simulink model "closed_loop"  (R2020a)
settings: Solver=ode45  StartTime=0.0  StopTime=10.0  RelTol=1e-3
values from neighbouring files (symbols this model uses):
  K = K8    [main.m]
  Kd = 1    [main.m]
  p = 4*N(i,j)-R1p    [h2AG.m]    (also in h2AS.m = 4*ns-R1p; parameters.mat = ; set_parameters.m = para)
undefined symbols (not defined in the file or in its folder): magnitude, sigbuilder_block
settings Model: Creator=mecsh  LastModifiedBy=mecsh

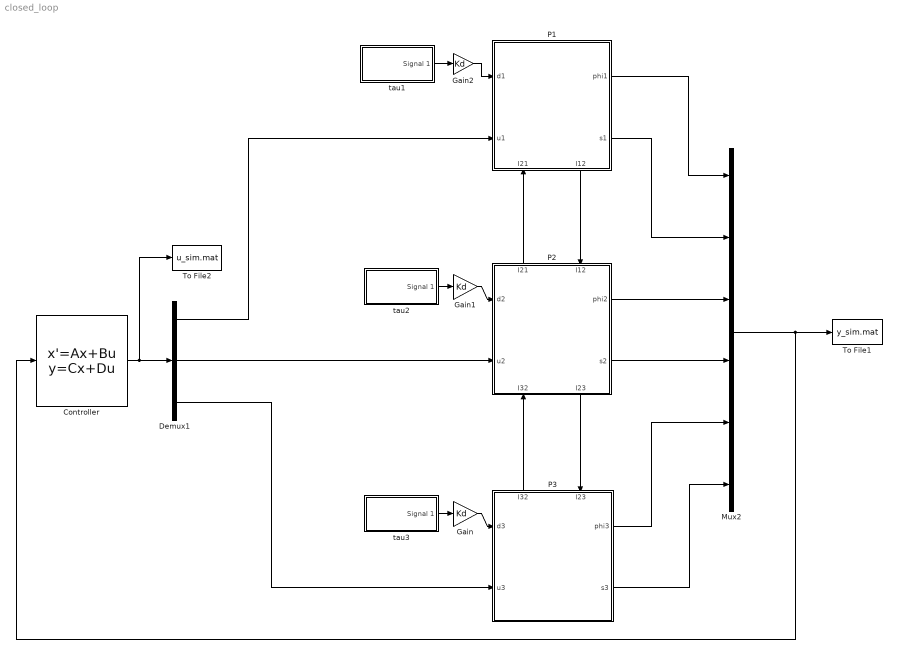
== system closed_loop ==
  Controller : StateSpace  A=K.A  B=K.B  C=K.C  D=K.D  InitialCondition=0
  Demux1 : Demux  Outputs=3
  Gain : Gain  Gain=Kd
  Gain1 : Gain  Gain=Kd
  Gain2 : Gain  Gain=Kd
  Mux2 : Mux  Inputs=6
  P1 : Subsystem
      settings: PortSchema="{\"entries\":[{\"content\":{\"sides\":[{\"content\":{\"connectorIds\":[\"In1\",\"In2\"]},\"type\":\"ConnectorPlacement.EquallySpacedRectSide\",\"uuid\":\"8ecf2bd6-8dd7-4624-a6b6-31e540f77a47\"},{\"content\":{\"connectorIds\":[\"Out1\",\"Out2\"],\"side\":\"RIGHT\"},\"type\":\"ConnectorPlacement.EquallySpacedRectSide\",\"uuid\":\"8430024e-b75d-4fb2-99a2-0065abf52074\"},{\"content\":{\"connectorIds\":[],\"side\":\"TOP\"},\"type\":\"ConnectorPlacement.EquallySpacedRectSide\",\"uuid\":\"c038c5bf-c588-4120-bde9-e57e7985113f\"},{\"content\":{\"connectorIds\":[\"In3\",\"Out3\"],\"side\":\"BOTTOM\"},\"type\":\"ConnectorPlacement.EquallySpacedRectSide\",\"uuid\":\"e08f6579-8c34-4bda-96ff-48e678e21df1\"}]},\"type\":\"ConnectorPlacement.EquallySpacedConnector\",\"uuid\":\"e152476a-752c-407e-9d79-b57d158a90de\"}],\"packageUris\":[\"http://schema.mathworks.com/mf0/Connector/19700101\"],\"version\":\"1.0\"}"
  P2 : Subsystem
      settings: PortSchema="{\"entries\":[{\"content\":{\"sides\":[{\"content\":{\"connectorIds\":[\"In1\",\"In2\"]},\"type\":\"ConnectorPlacement.EquallySpacedRectSide\",\"uuid\":\"4bcbf91d-3e1f-4b18-9cf2-1c48cd989a02\"},{\"content\":{\"connectorIds\":[\"Out1\",\"Out2\"],\"side\":\"RIGHT\"},\"type\":\"ConnectorPlacement.EquallySpacedRectSide\",\"uuid\":\"817b564b-dbb4-4a38-a63d-192f41fddb5e\"},{\"content\":{\"connectorIds\":[\"Out4\",\"In3\"],\"side\":\"TOP\"},\"type\":\"ConnectorPlacement.EquallySpacedRectSide\",\"uuid\":\"a66c876f-ee47-4f3c-90a0-c8c684866f46\"},{\"content\":{\"connectorIds\":[\"In4\",\"Out3\"],\"side\":\"BOTTOM\"},\"type\":\"ConnectorPlacement.EquallySpacedRectSide\",\"uuid\":\"ae0f9748-517d-4fb0-b861-7e671e2401a3\"}]},\"type\":\"ConnectorPlacement.EquallySpacedConnector\",\"uuid\":\"71628be4-01f7-4652-8912-34b5b1a2183b\"}],\"packageUris\":[\"http://schema.mathworks.com/mf0/Connector/19700101\"],\"version\":\"1.0\"}"
  P3 : Subsystem
      settings: PortSchema="{\"entries\":[{\"content\":{\"sides\":[{\"content\":{\"connectorIds\":[\"In1\",\"In2\"]},\"type\":\"ConnectorPlacement.EquallySpacedRectSide\",\"uuid\":\"4bcbf91d-3e1f-4b18-9cf2-1c48cd989a02\"},{\"content\":{\"connectorIds\":[\"Out1\",\"Out2\"],\"side\":\"RIGHT\"},\"type\":\"ConnectorPlacement.EquallySpacedRectSide\",\"uuid\":\"817b564b-dbb4-4a38-a63d-192f41fddb5e\"},{\"content\":{\"connectorIds\":[\"Out3\",\"In3\"],\"side\":\"TOP\"},\"type\":\"ConnectorPlacement.EquallySpacedRectSide\",\"uuid\":\"a66c876f-ee47-4f3c-90a0-c8c684866f46\"},{\"content\":{\"connectorIds\":[],\"side\":\"BOTTOM\"},\"type\":\"ConnectorPlacement.EquallySpacedRectSide\",\"uuid\":\"ae0f9748-517d-4fb0-b861-7e671e2401a3\"}]},\"type\":\"ConnectorPlacement.EquallySpacedConnector\",\"uuid\":\"71628be4-01f7-4652-8912-34b5b1a2183b\"}],\"packageUris\":[\"http://schema.mathworks.com/mf0/Connector/19700101\"],\"version\":\"1.0\"}"
  To File1 : ToFile  Filename=y_sim.mat  MatrixName=y_sim  SampleTime=0.01
  To File2 : ToFile  Filename=u_sim.mat  MatrixName=u_sim  SampleTime=0.01
  tau1 : Subsystem  Tag=STV Subsys  LoadFcn=sigbuilder_block('load');  StartFcn=sigbuilder_block('start');  StopFcn=sigbuilder_block('stop');  ClipboardFcn=sigbuilder_block('clipboard');  mask(Sigbuilder block){tuvar=[0:10]}
      mask help: Simulink:masks:SigbuilderBlock_MD
      mask init:
      | if ~strcmp(get_param(bdroot(gcbh),'SimulationStatus'),'stopped') tuvar = sigbuilder_block('maskInit'); end
      settings: CopyFcn=sigbuilder_block('copy');  DeleteFcn=sigbuilder_block('delete');  ModelCloseFcn=sigbuilder_block('modelClose');  PreSaveFcn=sigbuilder_block('preSave');  PauseFcn=sigbuilder_block('pause');  ContinueFcn=sigbuilder_block('continue');  NameChangeFcn=sigbuilder_block('namechange');  OpenFcn=sigbuilder_block('open',[437.6 199.2 550.4 400 ]);  CloseFcn=sigbuilder_block('close');
      mask Display: plot(0, 0, 100, 100,[2, 2, 32, 32, 2], [68, 8, 8, 68, 68],[32, 2], [38, 38], [32, 19, 2],[53, 60, 44], [32, 17, 17, 2],[16, 16, 31, 31]);txt = getActiveGroup(gcbh);text(2, 100, txt,'verticalAlignment', 'top');
  tau2 : Subsystem  Tag=STV Subsys  LoadFcn=sigbuilder_block('load');  StartFcn=sigbuilder_block('start');  StopFcn=sigbuilder_block('stop');  ClipboardFcn=sigbuilder_block('clipboard');  mask(Sigbuilder block){tuvar=[0:10]}
      mask help: Simulink:masks:SigbuilderBlock_MD
      mask init:
      | if ~strcmp(get_param(bdroot(gcbh),'SimulationStatus'),'stopped') tuvar = sigbuilder_block('maskInit'); end
      settings: CopyFcn=sigbuilder_block('copy');  DeleteFcn=sigbuilder_block('delete');  ModelCloseFcn=sigbuilder_block('modelClose');  PreSaveFcn=sigbuilder_block('preSave');  PauseFcn=sigbuilder_block('pause');  ContinueFcn=sigbuilder_block('continue');  NameChangeFcn=sigbuilder_block('namechange');  OpenFcn=sigbuilder_block('open',[437.6 199.2 550.4 400 ]);  CloseFcn=sigbuilder_block('close');
      mask Display: plot(0, 0, 100, 100,[2, 2, 32, 32, 2], [68, 8, 8, 68, 68],[32, 2], [38, 38], [32, 19, 2],[53, 60, 44], [32, 17, 17, 2],[16, 16, 31, 31]);txt = getActiveGroup(gcbh);text(2, 100, txt,'verticalAlignment', 'top');
  tau3 : Subsystem  Tag=STV Subsys  LoadFcn=sigbuilder_block('load');  StartFcn=sigbuilder_block('start');  StopFcn=sigbuilder_block('stop');  ClipboardFcn=sigbuilder_block('clipboard');  mask(Sigbuilder block){tuvar=[0:10]}
      mask help: Simulink:masks:SigbuilderBlock_MD
      mask init:
      | if ~strcmp(get_param(bdroot(gcbh),'SimulationStatus'),'stopped') tuvar = sigbuilder_block('maskInit'); end
      settings: CopyFcn=sigbuilder_block('copy');  DeleteFcn=sigbuilder_block('delete');  ModelCloseFcn=sigbuilder_block('modelClose');  PreSaveFcn=sigbuilder_block('preSave');  PauseFcn=sigbuilder_block('pause');  ContinueFcn=sigbuilder_block('continue');  NameChangeFcn=sigbuilder_block('namechange');  OpenFcn=sigbuilder_block('open',[437.6 199.2 550.4 400 ]);  CloseFcn=sigbuilder_block('close');
      mask Display: plot(0, 0, 100, 100,[2, 2, 32, 32, 2], [68, 8, 8, 68, 68],[32, 2], [38, 38], [32, 19, 2],[53, 60, 44], [32, 17, 17, 2],[16, 16, 31, 31]);txt = getActiveGroup(gcbh);text(2, 100, txt,'verticalAlignment', 'top');
  wires:
  P2/4(I21) -> P1/3(I21)
  P1/3(I12) -> P2/3(I12)
  P3/3(I32) -> P2/4(I32)
  P2/3(I23) -> P3/3(I23)
  P2/1(phi2) -> Mux2/3
  P2/2(s2) -> Mux2/4
  P1/1(phi1) -> Mux2/1
  P1/2(s1) -> Mux2/2
  P3/1(phi3) -> Mux2/5
  P3/2(s3) -> Mux2/6
  Mux2/1 -> To File1/1, Controller/1
  tau1/1(Signal 1) -> Gain2/1
  Controller/1 -> To File2/1, Demux1/1
  tau2/1(Signal 1) -> Gain1/1
  tau3/1(Signal 1) -> Gain/1
  Gain/1 -> P3/1(d3)
  Gain1/1 -> P2/1(d2)
  Gain2/1 -> P1/1(d1)
  Demux1/1 -> P1/2(u1)
  Demux1/2 -> P2/2(u2)
  Demux1/3 -> P3/2(u3)

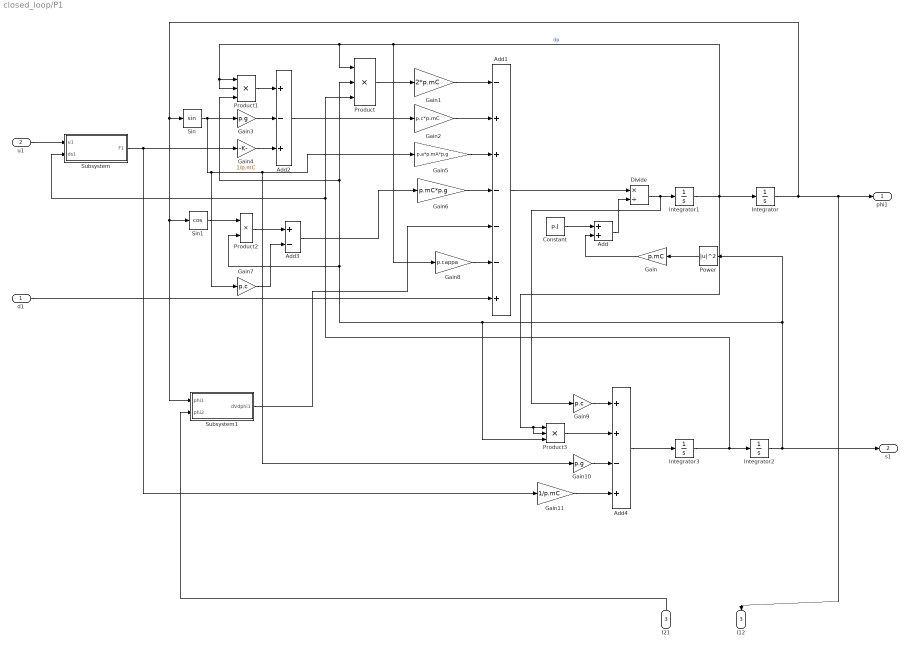
== system closed_loop/P1 ==
  d1 : Inport
  u1 : Inport  Port=2
  I21 : Inport  Port=3
  Add : Sum
  Add1 : Sum  Inputs=-++---+
  Add2 : Sum  Inputs=+-+
  Add3 : Sum  Inputs=+-
  Add4 : Sum  Inputs=++-+
  Constant : Constant  Value=p.J
  Divide : Product  Inputs=*/
  Gain : Gain  Gain=p.mC
  Gain1 : Gain  Gain=2*p.mC
  Gain10 : Gain  Gain=p.g
  Gain11 : Gain  Gain=1/p.mC
  Gain2 : Gain  Gain=p.c*p.mC
  Gain3 : Gain  Gain=p.g
  Gain4 : Gain  Gain=1/p.mC
  Gain5 : Gain  Gain=p.a*p.mA*p.g
  Gain6 : Gain  Gain=p.mC*p.g
  Gain7 : Gain  Gain=p.c
  Gain8 : Gain  Gain=p.cappa
  Gain9 : Gain  Gain=p.c
  Integrator{,1..3} (4 alike) : Integrator
  Power : Math  Operator=magnitude^2  SaturateOnIntegerOverflow=on
  Product : Product  Inputs=3
  Product1 : Product  Inputs=3
  Product2 : Product
  Product3 : Product  Inputs=3
  Sin : Trigonometry
  Sin1 : Trigonometry  Operator=cos
  Subsystem : Subsystem
  Subsystem1 : Subsystem
  phi1 : Outport
  s1 : Outport  Port=2
  I12 : Outport  Port=3
  wires:
  Integrator1/1 -> Product3/2, Product3/1, Gain8/1, Product1/2, Product1/1, Product/1, Integrator/1  "dp"
  Integrator3/1 -> Subsystem/2(ds1), Product/3, Integrator2/1
  Divide/1 -> Gain9/1, Integrator1/1
  Add/1 -> Divide/2
  Constant/1 -> Add/1
  Integrator2/1 -> Product3/3, Product2/2, Product1/3, Product/2, Power/1, s1/1
  Integrator/1 -> Subsystem1/1(phi1), Sin1/1, Sin/1, I12/1, phi1/1
  Power/1 -> Gain/1
  Gain/1 -> Add/2
  Add1/1 -> Divide/1
  Gain1/1 -> Add1/1
  Product/1 -> Gain1/1
  Gain2/1 -> Add1/2
  Add2/1 -> Gain2/1
  Product1/1 -> Add2/1
  Gain3/1 -> Add2/2
  Sin/1 -> Gain5/1, Gain10/1, Gain7/1, Gain3/1
  Gain4/1 -> Add2/3
  u1/1 -> Subsystem/1(u1)
  Gain5/1 -> Add1/3
  Gain6/1 -> Add1/4
  Add3/1 -> Gain6/1
  Product2/1 -> Add3/1
  Sin1/1 -> Product2/1
  Gain7/1 -> Add3/2
  Subsystem1/1(dVdphi1) -> Add1/5
  I21/1 -> Subsystem1/2(phi2)
  Gain8/1 -> Add1/6
  d1/1 -> Add1/7
  Add4/1 -> Integrator3/1
  Gain9/1 -> Add4/1
  Product3/1 -> Add4/2
  Gain10/1 -> Add4/3
  Gain11/1 -> Add4/4
  Subsystem/1(F1) -> Gain11/1, Gain4/1

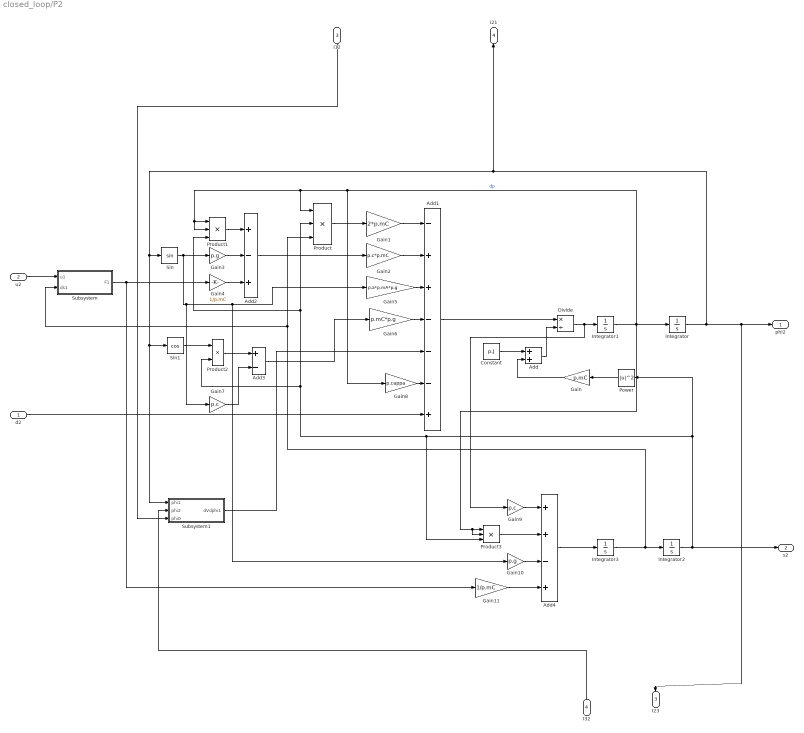
== system closed_loop/P2 ==
  d2 : Inport
  u2 : Inport  Port=2
  I12 : Inport  Port=3
  I32 : Inport  Port=4
  Add : Sum
  Add1 : Sum  Inputs=-++---+
  Add2 : Sum  Inputs=+-+
  Add3 : Sum  Inputs=+-
  Add4 : Sum  Inputs=++-+
  Constant : Constant  Value=p.J
  Divide : Product  Inputs=*/
  Gain : Gain  Gain=p.mC
  Gain1 : Gain  Gain=2*p.mC
  Gain10 : Gain  Gain=p.g
  Gain11 : Gain  Gain=1/p.mC
  Gain2 : Gain  Gain=p.c*p.mC
  Gain3 : Gain  Gain=p.g
  Gain4 : Gain  Gain=1/p.mC
  Gain5 : Gain  Gain=p.a*p.mA*p.g
  Gain6 : Gain  Gain=p.mC*p.g
  Gain7 : Gain  Gain=p.c
  Gain8 : Gain  Gain=p.cappa
  Gain9 : Gain  Gain=p.c
  Integrator{,1..3} (4 alike) : Integrator
  Power : Math  Operator=magnitude^2  SaturateOnIntegerOverflow=on
  Product : Product  Inputs=3
  Product1 : Product  Inputs=3
  Product2 : Product
  Product3 : Product  Inputs=3
  Sin : Trigonometry
  Sin1 : Trigonometry  Operator=cos
  Subsystem : Subsystem
  Subsystem1 : Subsystem
  phi2 : Outport
  s2 : Outport  Port=2
  I23 : Outport  Port=3
  I21 : Outport  Port=4
  wires:
  Gain11/1 -> Add4/4
  Add4/1 -> Integrator3/1
  Sin1/1 -> Product2/1
  Subsystem1/1(dVdphi1) -> Add1/5
  Gain9/1 -> Add4/1
  u2/1 -> Subsystem/1(u1)
  Divide/1 -> Gain9/1, Integrator1/1
  Integrator/1 -> I21/1, Subsystem1/1(phi1), Sin1/1, Sin/1, phi2/1, I23/1
  Subsystem/1(F1) -> Gain11/1, Gain4/1
  Gain7/1 -> Add3/2
  Gain6/1 -> Add1/4
  Product/1 -> Gain1/1
  Product1/1 -> Add2/1
  Add2/1 -> Gain2/1
  Integrator3/1 -> Subsystem/2(ds1), Product/3, Integrator2/1
  Integrator2/1 -> s2/1, Product3/3, Product2/2, Product1/3, Product/2, Power/1
  Gain2/1 -> Add1/2
  Gain1/1 -> Add1/1
  Gain4/1 -> Add2/3
  Constant/1 -> Add/1
  Integrator1/1 -> Product3/2, Product3/1, Gain8/1, Product1/2, Product1/1, Product/1, Integrator/1  "dp"
  Add/1 -> Divide/2
  I32/1 -> Subsystem1/2(phi2)
  Power/1 -> Gain/1
  Product2/1 -> Add3/1
  Add3/1 -> Gain6/1
  Add1/1 -> Divide/1
  Gain3/1 -> Add2/2
  Gain5/1 -> Add1/3
  Gain10/1 -> Add4/3
  Gain/1 -> Add/2
  Sin/1 -> Gain5/1, Gain10/1, Gain7/1, Gain3/1
  d2/1 -> Add1/7
  Gain8/1 -> Add1/6
  Product3/1 -> Add4/2
  I12/1 -> Subsystem1/3(phi0)

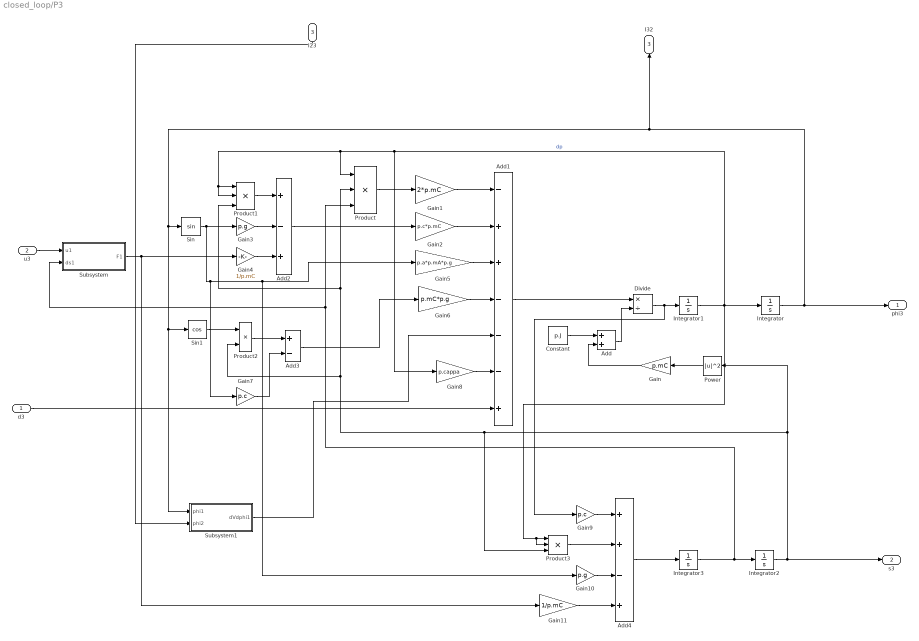
== system closed_loop/P3 ==
  d3 : Inport
  u3 : Inport  Port=2
  I23 : Inport  Port=3
  Add : Sum
  Add1 : Sum  Inputs=-++---+
  Add2 : Sum  Inputs=+-+
  Add3 : Sum  Inputs=+-
  Add4 : Sum  Inputs=++-+
  Constant : Constant  Value=p.J
  Divide : Product  Inputs=*/
  Gain : Gain  Gain=p.mC
  Gain1 : Gain  Gain=2*p.mC
  Gain10 : Gain  Gain=p.g
  Gain11 : Gain  Gain=1/p.mC
  Gain2 : Gain  Gain=p.c*p.mC
  Gain3 : Gain  Gain=p.g
  Gain4 : Gain  Gain=1/p.mC
  Gain5 : Gain  Gain=p.a*p.mA*p.g
  Gain6 : Gain  Gain=p.mC*p.g
  Gain7 : Gain  Gain=p.c
  Gain8 : Gain  Gain=p.cappa
  Gain9 : Gain  Gain=p.c
  Integrator{,1..3} (4 alike) : Integrator
  Power : Math  Operator=magnitude^2  SaturateOnIntegerOverflow=on
  Product : Product  Inputs=3
  Product1 : Product  Inputs=3
  Product2 : Product
  Product3 : Product  Inputs=3
  Sin : Trigonometry
  Sin1 : Trigonometry  Operator=cos
  Subsystem : Subsystem
  Subsystem1 : Subsystem
  phi3 : Outport
  s3 : Outport  Port=2
  I32 : Outport  Port=3
  wires:
  Gain11/1 -> Add4/4
  Add4/1 -> Integrator3/1
  Sin1/1 -> Product2/1
  Subsystem1/1(dVdphi1) -> Add1/5
  Gain9/1 -> Add4/1
  Divide/1 -> Gain9/1, Integrator1/1
  Integrator/1 -> I32/1, Subsystem1/1(phi1), Sin1/1, Sin/1, phi3/1
  Subsystem/1(F1) -> Gain11/1, Gain4/1
  Gain7/1 -> Add3/2
  Gain6/1 -> Add1/4
  Product/1 -> Gain1/1
  Product1/1 -> Add2/1
  Add2/1 -> Gain2/1
  Integrator3/1 -> Subsystem/2(ds1), Product/3, Integrator2/1
  Integrator2/1 -> s3/1, Product3/3, Product2/2, Product1/3, Product/2, Power/1
  Gain2/1 -> Add1/2
  Gain1/1 -> Add1/1
  Gain4/1 -> Add2/3
  Constant/1 -> Add/1
  Integrator1/1 -> Product3/2, Product3/1, Gain8/1, Product1/2, Product1/1, Product/1, Integrator/1  "dp"
  Add/1 -> Divide/2
  Power/1 -> Gain/1
  Product2/1 -> Add3/1
  Add3/1 -> Gain6/1
  Add1/1 -> Divide/1
  Gain3/1 -> Add2/2
  Gain5/1 -> Add1/3
  Gain10/1 -> Add4/3
  Gain/1 -> Add/2
  Sin/1 -> Gain5/1, Gain10/1, Gain7/1, Gain3/1
  d3/1 -> Add1/7
  Gain8/1 -> Add1/6
  Product3/1 -> Add4/2
  u3/1 -> Subsystem/1(u1)
  I23/1 -> Subsystem1/2(phi2)

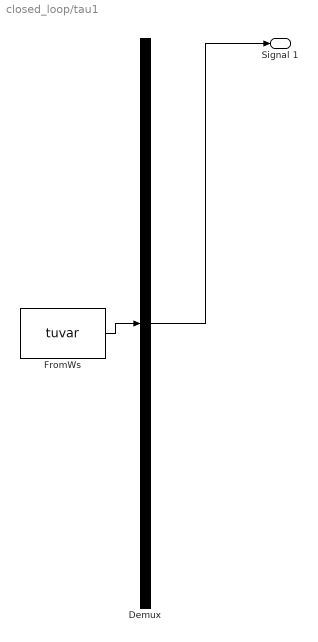
== system closed_loop/tau1 ==
  Demux : Demux  Tag=STV Demux  Outputs=1
      settings: DisplayOption=none
  FromWs : FromWorkspace  Tag=STV FromWs  VariableName=tuvar
      SigBuilderData=|
      | common.afterFinalStr = 'Extrapolate'
      | common.sampleTime = 0
      | dataSet.timeRange = [0 10]
      | dataSet.name = 'Group 1'
      | sbobj.Groups.Name = 'Group 1'
      | sbobj.Groups.Signals.Name = 'Signal 1'
      | sbobj.Groups.Signals.XData = [0 1 1 1.5 1.5 10]
      | sbobj.Groups.Signals.YData = [0 0 0.5 0.5 0 0]
  Signal 1 : Outport  Tag=STV Outport  VectorParamsAs1DForOutWhenUnconnected=off
  wires:
  Demux/1 -> Signal 1/1
  FromWs/1 -> Demux/1

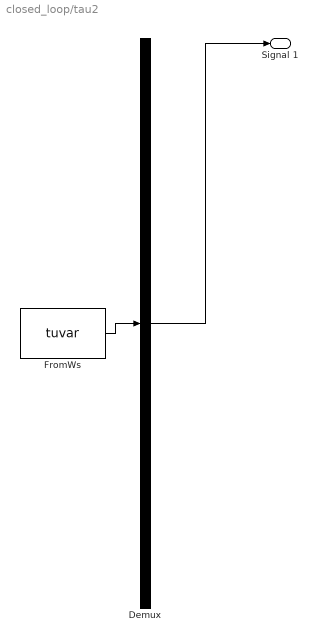
== system closed_loop/tau2 ==
  Demux : Demux  Tag=STV Demux  Outputs=1
      settings: DisplayOption=none
  FromWs : FromWorkspace  Tag=STV FromWs  VariableName=tuvar
      SigBuilderData=|
      | common.afterFinalStr = 'Extrapolate'
      | common.sampleTime = 0
      | dataSet.timeRange = [0 10]
      | dataSet.name = 'Group 1'
      | sbobj.Groups.Name = 'Group 1'
      | sbobj.Groups.Signals.Name = 'Signal 1'
      | sbobj.Groups.Signals.XData = [0 1 1 1.5 1.5 10]
      | sbobj.Groups.Signals.YData = [0 0 -1 -1 0 0]
  Signal 1 : Outport  Tag=STV Outport  VectorParamsAs1DForOutWhenUnconnected=off
  wires:
  Demux/1 -> Signal 1/1
  FromWs/1 -> Demux/1

== system closed_loop/tau3 ==
  Demux : Demux  Tag=STV Demux  Outputs=1
      settings: DisplayOption=none
  FromWs : FromWorkspace  Tag=STV FromWs  VariableName=tuvar
      SigBuilderData=|
      | common.afterFinalStr = 'Extrapolate'
      | common.sampleTime = 0
      | dataSet.timeRange = [0 10]
      | dataSet.name = 'Group 1'
      | sbobj.Groups.Name = 'Group 1'
      | sbobj.Groups.Signals.Name = 'Signal 1'
      | sbobj.Groups.Signals.XData = [0 1 1 1.5 1.5 10]
      | sbobj.Groups.Signals.YData = [0 0 0.2 0.2 0 0]
  Signal 1 : Outport  Tag=STV Outport  VectorParamsAs1DForOutWhenUnconnected=off
  wires:
  Demux/1 -> Signal 1/1
  FromWs/1 -> Demux/1

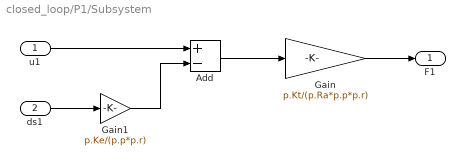
== system closed_loop/P1/Subsystem ==
  u1 : Inport
  ds1 : Inport  Port=2
  Add : Sum  Inputs=+-
  Gain : Gain  Gain=p.Kt/(p.Ra*p.p*p.r)
  Gain1 : Gain  Gain=p.Ke/(p.p*p.r)
  F1 : Outport
  wires:
  Gain/1 -> F1/1
  Add/1 -> Gain/1
  u1/1 -> Add/1
  ds1/1 -> Gain1/1
  Gain1/1 -> Add/2

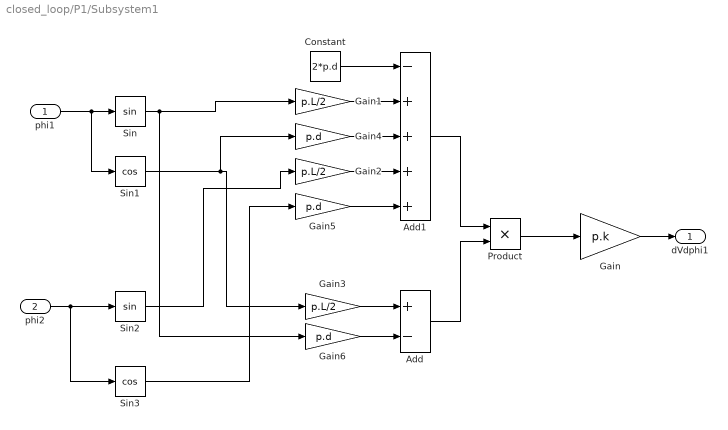
== system closed_loop/P1/Subsystem1 ==
  phi1 : Inport
  phi2 : Inport  Port=2
  Add : Sum  Inputs=+-
  Add1 : Sum  Inputs=-++++
  Constant : Constant  Value=2*p.d
  Gain : Gain  Gain=p.k
  Gain1 : Gain  Gain=p.L/2
  Gain2 : Gain  Gain=p.L/2
  Gain3 : Gain  Gain=p.L/2
  Gain4 : Gain  Gain=p.d
  Gain5 : Gain  Gain=p.d
  Gain6 : Gain  Gain=p.d
  Product : Product
  Sin : Trigonometry
  Sin1 : Trigonometry  Operator=cos
  Sin2 : Trigonometry
  Sin3 : Trigonometry  Operator=cos
  dVdphi1 : Outport
  wires:
  Gain/1 -> dVdphi1/1
  Product/1 -> Gain/1
  Add/1 -> Product/2
  Add1/1 -> Product/1
  Constant/1 -> Add1/1
  phi1/1 -> Sin1/1, Sin/1
  phi2/1 -> Sin3/1, Sin2/1
  Gain1/1 -> Add1/2
  Gain2/1 -> Add1/4
  Gain3/1 -> Add/1
  Gain4/1 -> Add1/3
  Gain5/1 -> Add1/5
  Gain6/1 -> Add/2
  Sin/1 -> Gain6/1, Gain1/1
  Sin1/1 -> Gain3/1, Gain4/1
  Sin2/1 -> Gain2/1
  Sin3/1 -> Gain5/1

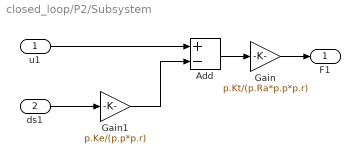
== system closed_loop/P2/Subsystem ==
  u1 : Inport
  ds1 : Inport  Port=2
  Add : Sum  Inputs=+-
  Gain : Gain  Gain=p.Kt/(p.Ra*p.p*p.r)
  Gain1 : Gain  Gain=p.Ke/(p.p*p.r)
  F1 : Outport
  wires:
  Gain/1 -> F1/1
  Add/1 -> Gain/1
  u1/1 -> Add/1
  ds1/1 -> Gain1/1
  Gain1/1 -> Add/2

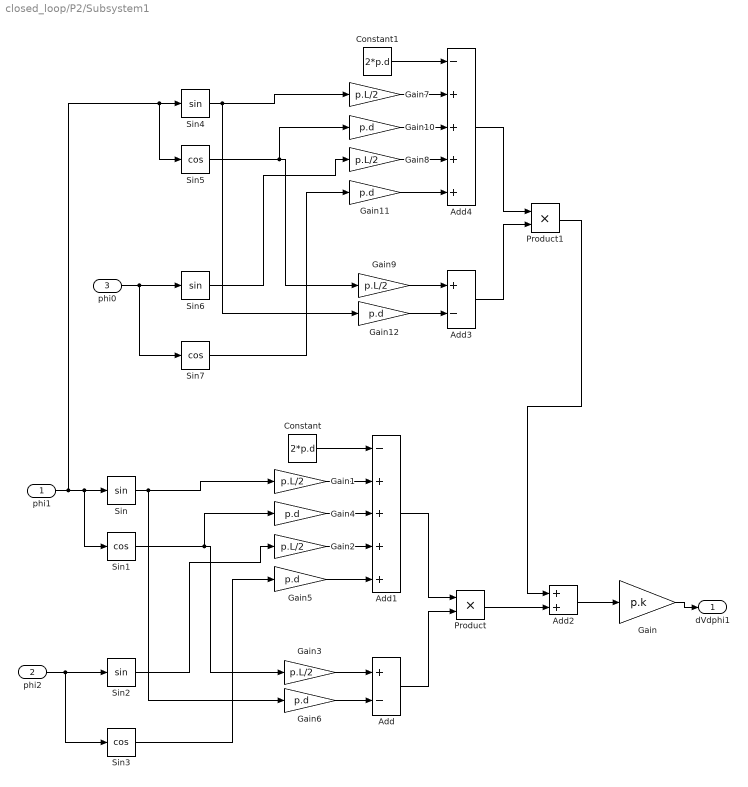
== system closed_loop/P2/Subsystem1 ==
  phi1 : Inport
  phi2 : Inport  Port=2
  phi0 : Inport  Port=3
  Add : Sum  Inputs=+-
  Add1 : Sum  Inputs=-++++
  Add2 : Sum
  Add3 : Sum  Inputs=+-
  Add4 : Sum  Inputs=-++++
  Constant : Constant  Value=2*p.d
  Constant1 : Constant  Value=2*p.d
  Gain : Gain  Gain=p.k
  Gain{1..3,7..9} (6 alike) : Gain  Gain=p.L/2
  Gain{4..6,10..12} (6 alike) : Gain  Gain=p.d
  Product : Product
  Product1 : Product
  Sin{,2,4,6} (4 alike) : Trigonometry
  Sin{1,3,5,7} (4 alike) : Trigonometry  Operator=cos
  dVdphi1 : Outport
  wires:
  Gain/1 -> dVdphi1/1
  Add/1 -> Product/2
  Add1/1 -> Product/1
  Constant/1 -> Add1/1
  phi2/1 -> Sin3/1, Sin2/1
  Gain1/1 -> Add1/2
  Gain2/1 -> Add1/4
  Gain3/1 -> Add/1
  Gain4/1 -> Add1/3
  Gain5/1 -> Add1/5
  Gain6/1 -> Add/2
  Sin/1 -> Gain6/1, Gain1/1
  Sin1/1 -> Gain3/1, Gain4/1
  Sin2/1 -> Gain2/1
  Sin3/1 -> Gain5/1
  Product/1 -> Add2/2
  Add2/1 -> Gain/1
  Add4/1 -> Product1/1
  Sin7/1 -> Gain11/1
  Sin6/1 -> Gain8/1
  Sin5/1 -> Gain9/1, Gain10/1
  Constant1/1 -> Add4/1
  Sin4/1 -> Gain12/1, Gain7/1
  Gain7/1 -> Add4/2
  Gain12/1 -> Add3/2
  Gain8/1 -> Add4/4
  Gain10/1 -> Add4/3
  Gain9/1 -> Add3/1
  phi0/1 -> Sin7/1, Sin6/1
  phi1/1 -> Sin5/1, Sin4/1, Sin1/1, Sin/1
  Add3/1 -> Product1/2
  Gain11/1 -> Add4/5
  Product1/1 -> Add2/1

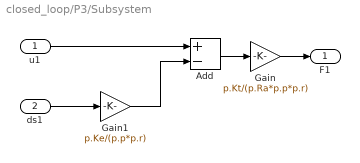
== system closed_loop/P3/Subsystem ==
  u1 : Inport
  ds1 : Inport  Port=2
  Add : Sum  Inputs=+-
  Gain : Gain  Gain=p.Kt/(p.Ra*p.p*p.r)
  Gain1 : Gain  Gain=p.Ke/(p.p*p.r)
  F1 : Outport
  wires:
  Gain/1 -> F1/1
  Add/1 -> Gain/1
  u1/1 -> Add/1
  ds1/1 -> Gain1/1
  Gain1/1 -> Add/2

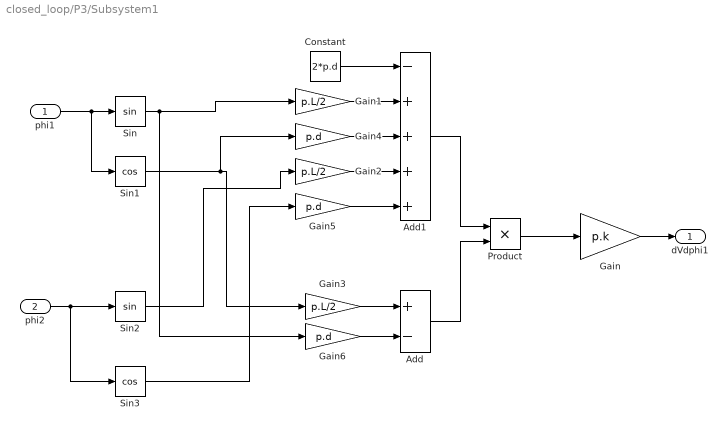
== system closed_loop/P3/Subsystem1 ==
  phi1 : Inport
  phi2 : Inport  Port=2
  Add : Sum  Inputs=+-
  Add1 : Sum  Inputs=-++++
  Constant : Constant  Value=2*p.d
  Gain : Gain  Gain=p.k
  Gain1 : Gain  Gain=p.L/2
  Gain2 : Gain  Gain=p.L/2
  Gain3 : Gain  Gain=p.L/2
  Gain4 : Gain  Gain=p.d
  Gain5 : Gain  Gain=p.d
  Gain6 : Gain  Gain=p.d
  Product : Product
  Sin : Trigonometry
  Sin1 : Trigonometry  Operator=cos
  Sin2 : Trigonometry
  Sin3 : Trigonometry  Operator=cos
  dVdphi1 : Outport
  wires:
  Gain/1 -> dVdphi1/1
  Product/1 -> Gain/1
  Add/1 -> Product/2
  Add1/1 -> Product/1
  Constant/1 -> Add1/1
  phi1/1 -> Sin1/1, Sin/1
  phi2/1 -> Sin3/1, Sin2/1
  Gain1/1 -> Add1/2
  Gain2/1 -> Add1/4
  Gain3/1 -> Add/1
  Gain4/1 -> Add1/3
  Gain5/1 -> Add1/5
  Gain6/1 -> Add/2
  Sin/1 -> Gain6/1, Gain1/1
  Sin1/1 -> Gain3/1, Gain4/1
  Sin2/1 -> Gain2/1
  Sin3/1 -> Gain5/1
